simulink model "valid_propagation_concept"  (R2023b)
settings: Solver=VariableStepAuto  StartTime=0.0  StopTime=10.0  RelTol=1e-3
libraries: hdlsllib x14, simulink x1
settings Model: Creator=foregan  LastModifiedBy=foregan

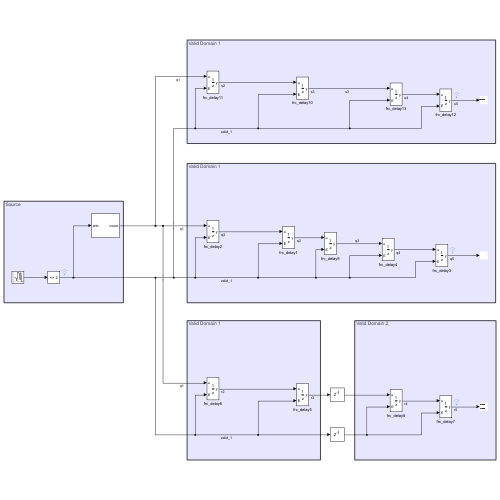
[thumbnail: Simulink's stored preview of the top-level diagram]
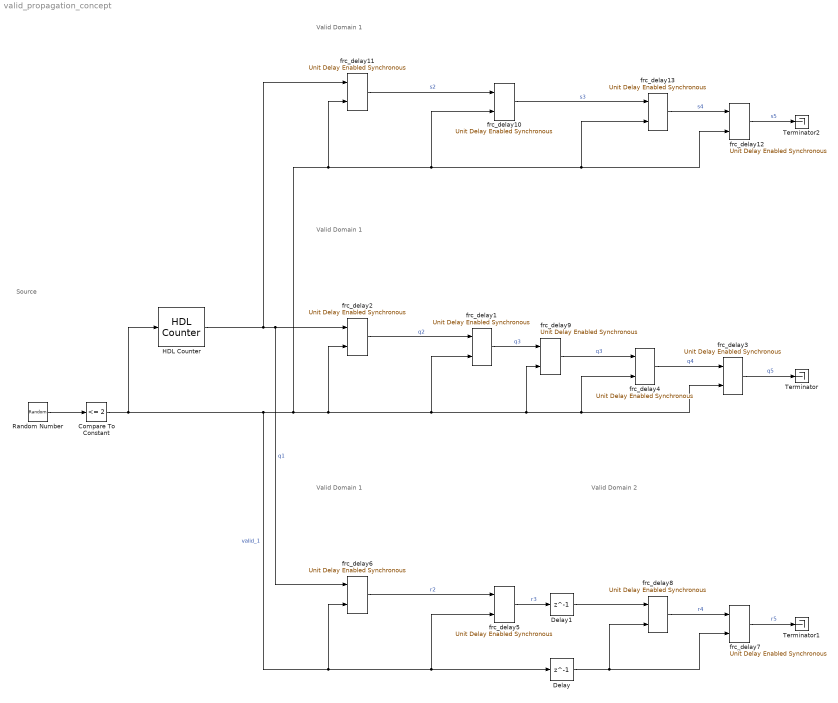
== system valid_propagation_concept ==
  note: Valid Domain 2
  note: Source
  note: Valid Domain 1
  note: Valid Domain 1
  note: Valid Domain 1
  Compare To Constant : simulink/Logic and Bit Operations/Compare To Constant  relop=<=  const=2  OutDataTypeStr=boolean
  Delay : Delay  DelayLength=1
  Delay1 : Delay  DelayLength=1
  HDL Counter : hdlsllib/Sources/HDL Counter  CountType=Count limited  CountInit=0  CountStep=1  CountMax=25  CountFromType=Initial value  CountFrom=0  CountResetPort=off  CountLoadPort=off  CountEnbPort=on  CountDirPort=off  CountHitOutputPort=off  CountDataType=Unsigned  CountWordLen=8  CountFracLen=0  CountSampTime=1
  Random Number : RandomNumber  Mean=0.5  SampleTime=0.1
  Terminator : Terminator
  Terminator1 : Terminator
  Terminator2 : Terminator
  frc_delay{1..13} (13 alike) : hdlsllib/Discrete/Unit Delay Enabled Synchronous  InitialCondition=0  SampleTime=-1
  wires:
  Random Number/1 -> Compare To Constant/1
  frc_delay2/1 -> frc_delay1/1  "q2"
  frc_delay9/1 -> frc_delay4/1  "q3"
  frc_delay4/1 -> frc_delay3/1  "q4"
  frc_delay3/1 -> Terminator/1  "q5"
  frc_delay7/1 -> Terminator1/1  "r5"
  frc_delay6/1 -> frc_delay5/1  "r2"
  frc_delay5/1 -> Delay1/1  "r3"
  frc_delay8/1 -> frc_delay7/1  "r4"
  Delay1/1 -> frc_delay8/1
  Delay/1 -> frc_delay8/2, frc_delay7/2
  frc_delay1/1 -> frc_delay9/1  "q3"
  Compare To Constant/1 -> frc_delay5/2, Delay/1, frc_delay6/2, frc_delay10/2, frc_delay13/2, frc_delay12/2, frc_delay11/2, frc_delay1/2, frc_delay9/2, frc_delay4/2, frc_delay3/2, frc_delay2/2, HDL Counter/1  "valid_1"
  frc_delay12/1 -> Terminator2/1  "s5"
  frc_delay11/1 -> frc_delay10/1  "s2"
  frc_delay10/1 -> frc_delay13/1  "s3"
  frc_delay13/1 -> frc_delay12/1  "s4"
  HDL Counter/1 -> frc_delay11/1, frc_delay6/1, frc_delay2/1  "q1"
